simulink model "nonlinear_model"  (R2021a)
settings: Solver=VariableStepAuto  StartTime=0.0  StopTime=10  RelTol=1e-3
libraries: RCTblocks x5, cstblocks x1
settings Model: Creator=MarcosRPesanteColón  LastModifiedBy=MarcosRPesanteColón

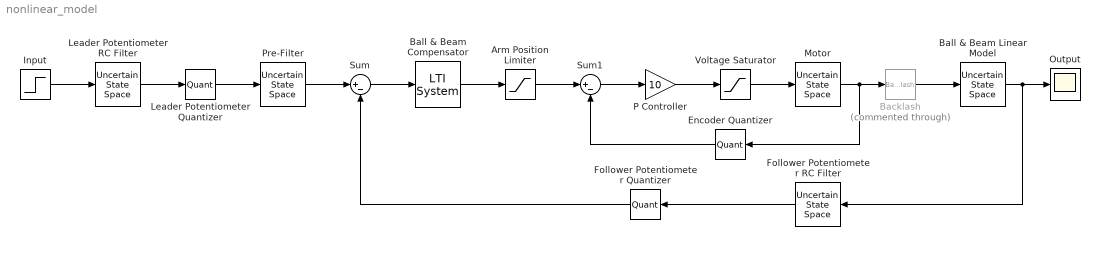
== system nonlinear_model ==
  Arm Position Limiter : Saturate  UpperLimit=pi/2  LowerLimit=-pi/2
  Backlash : Backlash  Commented=through  BacklashWidth=2*pi/4096
  Ball & Beam Compensator : cstblocks/LTI System  sys=G_c  IC=[]
  Ball & Beam Linear Model : RCTblocks/Uncertain State Space  Tag=USS  USystem=G_bb  UValue=[]  X0=[]  uX0=[]
      settings: SourceProductBaseCode=RC
  Encoder Quantizer : Quantizer  QuantizationInterval=pi/2048
  Follower Potentiometer Quantizer : Quantizer  QuantizationInterval=0.4255/4096
  Follower Potentiometer RC Filter : RCTblocks/Uncertain State Space  Tag=USS  USystem=G_f  UValue=[]  X0=[]  uX0=[]
      settings: SourceProductBaseCode=RC
  Input : Step  SampleTime=0
  Leader Potentiometer Quantizer : Quantizer  QuantizationInterval=0.4255/4096
  Leader Potentiometer RC Filter : RCTblocks/Uncertain State Space  Tag=USS  USystem=G_l  UValue=[]  X0=[]  uX0=[]
      settings: SourceProductBaseCode=RC
  Motor : RCTblocks/Uncertain State Space  Tag=USS  USystem=G_m_tilde  UValue=[]  X0=[]  uX0=[]
      settings: SourceProductBaseCode=RC
  Output : Scope
  P Controller : Gain  Gain=10
  Pre-Filter : RCTblocks/Uncertain State Space  Tag=USS  USystem=G_f  UValue=[]  X0=[]  uX0=[]
      settings: SourceProductBaseCode=RC
  Sum : Sum  Inputs=|+-
  Sum1 : Sum  Inputs=|+-
  Voltage Saturator : Saturate  UpperLimit=5  LowerLimit=-5
  wires:
  Sum1/1 -> P Controller/1
  P Controller/1 -> Voltage Saturator/1
  Sum/1 -> Ball & Beam Compensator/1
  Ball & Beam Linear Model/1 -> Output/1, Follower Potentiometer RC Filter/1
  Voltage Saturator/1 -> Motor/1
  Encoder Quantizer/1 -> Sum1/2
  Follower Potentiometer Quantizer/1 -> Sum/2
  Motor/1 -> Backlash/1, Encoder Quantizer/1
  Ball & Beam Compensator/1 -> Arm Position Limiter/1
  Arm Position Limiter/1 -> Sum1/1
  Leader Potentiometer Quantizer/1 -> Pre-Filter/1
  Follower Potentiometer RC Filter/1 -> Follower Potentiometer Quantizer/1
  Input/1 -> Leader Potentiometer RC Filter/1
  Leader Potentiometer RC Filter/1 -> Leader Potentiometer Quantizer/1
  Pre-Filter/1 -> Sum/1
  Backlash/1 -> Ball & Beam Linear Model/1
